simulink model "tqdtqr_rebuild_V3"  (R2021b)
settings: Solver=VariableStepAuto  StartTime=0.0  StopTime=10.0  RelTol=1e-3
undefined symbols (not defined in the file): ATQD_AfterTqMinGain_X_Deg, ATQD_APSCreepBaseTqD_X_kph, ATQD_APSCreepBaseTqD_Y_Deg, ATQD_APSCreepBaseTqR_X_kph, ATQD_APSCreepBaseTqR_Y_Deg, ATQD_APSCreepIterm_X_kph, ATQD_APSCreepIterm_Y_kph, ATQD_APSCreepPterm_X_kph, ATQD_APSCreepPterm_Y_kph, ATQD_APSDecReq_X_kph, ATQD_APSDecReq_Y_mps2, ATQD_APSDecReqCMD_X_kph, ATQD_APSDecReqTs_X_pct, ATQD_APSDecTimeGain_X_Deg, ATQD_APSDecTimeGain_Y_s, ATQD_APSReqLowSpd_X_Deg, ATQD_AutoHoldReleaseBPS_X_Deg, ATQD_AWDLoadTrqnsGain_X_kg, ATQD_AWDLoadTrqnsGain_Y_pct, ATQD_BOSEnBPSPosn_X_kph, ATQD_BOSMap_X_rpm, ATQD_BOSMap_Y_pct, ATQD_CreepBaseTqD_X_kph, ATQD_CreepBaseTqD_Y_Deg, ATQD_CreepBaseTqR_X_kph, ATQD_CreepBaseTqR_Y_Deg, ATQD_CreepBPSDisPosn_X_Deg, ATQD_CreepBPSDisPosnR_X_Deg, ATQD_CreepBPSEnPosn_X_Deg, ATQD_CreepBPSEnPosnR_X_Deg, ATQD_CreepDeltaTq_X_kph, ATQD_CreepIterm_X_kph, ATQD_CreepIterm_Y_kph, ATQD_CreepItermMaxLimit_X_pct, ATQD_CreepPreloadTime_X_kph, ATQD_CreepPreloadTq_X_kph, ATQD_CreepPreloadTq_Y_s, ATQD_CreepProtTq_X_Deg, ATQD_CreepPterm_X_kph, ATQD_CreepPterm_Y_kph, ATQD_CreepRrTqSpRat_X_rpm, ATQD_CreepRrTqSpRat_Y_Nm, ATQD_CreepTargetSpdD_X_pct, ATQD_CreepTargetSpdR_X_pct, ATQD_CreepUpLimitTq_X_rpm, ATQD_DecIneOPDHoldEnDelay_X_Deg, ATQD_DecIneOPDHoldEnDelay_Y_bar, ATQD_ECOTqMapD_X_rpm, ATQD_ECOTqMapD_Y_pct, ATQD_EMTqMapD_X_rpm, ATQD_EMTqMapD_Y_pct, ATQD_EOPDTqMapDCon_X_rpm, ATQD_EOPDTqMapDCon_Y_Deg, ATQD_EstInitVehWeight_X_c, ATQD_FAfterTqCMDGain_X_rpm, ATQD_FAfterTqCMDGain_Y_pct, ATQD_ForceLowSpd_X_Deg, ATQD_ForcePLimitSpd_X_Deg, ATQD_FrLossMAPLowV_X_rpm, ATQD_FrLossMAPLowV_Y_Nm ... (+949)
libraries: simulink x235, hcu_lib x208, tqr x63, tqd x6
(part 11 of 37)

== system tqdtqr_rebuild_V3/Input_Convert/Main function/Front//Rear zero point transfer ==
  note: Determine increase/decrease value
  note: Detemine rear zero transform
  note: Rear zero up/low boundary
  note: Detemine front zero transform
  note: Front zero up/low boundary
  BSCPIn_outputs : Inport
  BSignalConvert_outputs : Inport  Port=2
  BMain_outputs : Inport  Port=3
  VTQD_CreepPrLoadEnable_flg : Inport  Port=4
  VTQD_PreLoadPreEn_flg : Inport  Port=5
  AND : Logic  Inputs=4  AllPortsSameDT=off  OutDataTypeStr=boolean
  AND1 : Logic  Inputs=4  AllPortsSameDT=off  OutDataTypeStr=boolean
  Bus Selector : BusSelector  OutputSignals=VVMC_ADASActive_flg,VVMC_ACCPedalOvrd_flg,VVMC_EstSlope_Deg,VINP_VehSpeed_kph
  Bus Selector1 : BusSelector  OutputSignals=VTQR_EVDriveMode_enum,VTQD_TqTargetShaftSpd_rpm,VTQR_LaunchEn_flg,VTQD_RegenMode_enum
  Bus Selector2 : BusSelector  OutputSignals=VTQD_AfterAvailableTqDemFr_Nm,VTQD_AfterAvailableTqDemRr_Nm,VTQR_FEDUWhlTqReqSmoothDelay_Nm,VTQR_REDUWhlTqReqSmoothDelay_Nm
  Constant : Constant  Value=ZERO_FLOAT
  Constant{1,11,13..14} (4 alike) : Constant  Value=ENUM_DRIVEMODE_ECO
  Constant10 : Constant  Value=KTQR_OPDNoZeroTransSpd_kph
  Constant{2,12,15,18} (4 alike) : Constant  Value=ENUM_DRIVEMODE_NRM
  Constant{3,16..17,19} (4 alike) : Constant  Value=ENUM_DRIVEMODE_SPORT
  Constant20 : Constant  Value=ZERO_FLOAT
  Constant{4,21,28..29} (4 alike) : Constant  Value=ENUM_TQZEROTRANS_POSITIVE
  Constant22 : Constant  Value=ENUM_TQZEROTRANS_NEGATIVE
  Constant23 : Constant  Value=ENUM_TQZEROTRANS_NOZEROTRANS
  Constant24 : Constant  Value=KTQR_CreepZeroTransSW_flg
  Constant25 : Constant  Value=ENUM_REGENLEVEL_OPD
  Constant26 : Constant  Value=KTQR_OPDNoZeroTransTq_Nm
  Constant27 : Constant  Value=KTQR_OPDNoZeroTransSpd_kph
  Constant5 : Constant  Value=ENUM_TQZEROTRANS_NEGATIVE
  Constant6 : Constant  Value=ENUM_TQZEROTRANS_NOZEROTRANS
  Constant7 : Constant  Value=KTQR_CreepZeroTransSW_flg
  Constant8 : Constant  Value=ENUM_REGENLEVEL_OPD
  Constant9 : Constant  Value=KTQR_OPDNoZeroTransTq_Nm
  EcoLow : tqr/TQR/Determine Torque Request/TorqueArbitrament/TorqueSmooth/Front Torque zero point transfer boundary map/EcoLow  SystemSampleTime=-1  VariantActivationTime=update diagram  Latency=0  AutoFrameSizeCalculation=off
  EcoLow1 : tqr/TQR/Determine Torque Request/TorqueArbitrament/TorqueSmooth/Rear Torque zero point transfer boundary map/EcoLow  SystemSampleTime=-1  VariantActivationTime=update diagram  Latency=0  AutoFrameSizeCalculation=off
  EcoUP : tqr/TQR/Determine Torque Request/TorqueArbitrament/TorqueSmooth/Front Torque zero point transfer boundary map/EcoUP  SystemSampleTime=-1  VariantActivationTime=update diagram  Latency=0  AutoFrameSizeCalculation=off
  EcoUP1 : tqr/TQR/Determine Torque Request/TorqueArbitrament/TorqueSmooth/Rear Torque zero point transfer boundary map/EcoUP  SystemSampleTime=-1  VariantActivationTime=update diagram  Latency=0  AutoFrameSizeCalculation=off
  Equal{,1..13} (14 alike) : RelationalOperator  Operator===  OutDataTypeStr=boolean  RndMeth=Simplest
  If{1..4} (4 alike) : If  NumInputs=3  IfExpression=u1~= 0  ElseIfExpressions=u2 ~= 0, u3 ~=0  ShowElse=off
  Logical Operator : Logic  Inputs=7  AllPortsSameDT=off  OutDataTypeStr=boolean
  Logical Operator{1..4,6..9} (8 alike) : Logic  Operator=NOT  AllPortsSameDT=off  OutDataTypeStr=boolean
  Logical Operator5 : Logic  Inputs=7  AllPortsSameDT=off  OutDataTypeStr=boolean
  Merge{,1..3} (4 alike) : Merge  Inputs=3
  NOT{,1..3} (4 alike) : Logic  Operator=NOT  AllPortsSameDT=off  OutDataTypeStr=boolean
  Negative Rate limit Determination : Subsystem  TreatAsAtomicUnit=on
  Negative Rate limit Determination1 : Subsystem  AncestorBlock=tqr/TQR/Determine Torque Request/TorqueArbitrament/TorqueSmooth/Rear wheel rate limit determination/Negative Rate limit Determination  TreatAsAtomicUnit=on
  NormalLow : tqr/TQR/Determine Torque Request/TorqueArbitrament/TorqueSmooth/Front Torque zero point transfer boundary map/NormalLow  SystemSampleTime=-1  VariantActivationTime=update diagram  Latency=0  AutoFrameSizeCalculation=off
  NormalLow1 : tqr/TQR/Determine Torque Request/TorqueArbitrament/TorqueSmooth/Rear Torque zero point transfer boundary map/NormalLow  SystemSampleTime=-1  VariantActivationTime=update diagram  Latency=0  AutoFrameSizeCalculation=off
  NormalUP : tqr/TQR/Determine Torque Request/TorqueArbitrament/TorqueSmooth/Front Torque zero point transfer boundary map/NormalUP  SystemSampleTime=-1  VariantActivationTime=update diagram  Latency=0  AutoFrameSizeCalculation=off
  NormalUP1 : tqr/TQR/Determine Torque Request/TorqueArbitrament/TorqueSmooth/Rear Torque zero point transfer boundary map/NormalUP  SystemSampleTime=-1  VariantActivationTime=update diagram  Latency=0  AutoFrameSizeCalculation=off
  OR{,1..3} (4 alike) : Logic  Operator=OR  AllPortsSameDT=off  OutDataTypeStr=boolean
  Positive Rate limit Determination : Subsystem  TreatAsAtomicUnit=on
  Positive Rate limit Determination1 : Subsystem  TreatAsAtomicUnit=on
  Relational Operator : RelationalOperator  Operator=<  OutDataTypeStr=boolean  RndMeth=Simplest
  Relational Operator1 : RelationalOperator  Operator=>  OutDataTypeStr=boolean  RndMeth=Simplest
  Relational Operator10 : RelationalOperator  Operator===  OutDataTypeStr=boolean  RndMeth=Simplest
  Relational Operator11 : RelationalOperator  Operator===  OutDataTypeStr=boolean  RndMeth=Simplest
  Relational Operator2 : RelationalOperator  OutDataTypeStr=boolean  RndMeth=Simplest
  Relational Operator{3..4,8..9} (4 alike) : RelationalOperator  Operator=<=  OutDataTypeStr=boolean  RndMeth=Simplest
  Relational Operator5 : RelationalOperator  Operator=<  OutDataTypeStr=boolean  RndMeth=Simplest
  Relational Operator6 : RelationalOperator  Operator=>  OutDataTypeStr=boolean  RndMeth=Simplest
  Relational Operator7 : RelationalOperator  OutDataTypeStr=boolean  RndMeth=Simplest
  Relay1 : Relay  OnSwitchValue=KTQD_OPDHoldGradeUp_Deg  OffSwitchValue=KTQD_OPDHoldGradeDown_Deg  OutDataTypeStr=boolean
      settings: AttributesFormatString=|
      | On : %<OnSwitchValue>
      | Off : %<OffSwitchValue>
  Relay2 : Relay  OnSwitchValue=KTQD_OPDHoldGradeUp_Deg  OffSwitchValue=KTQD_OPDHoldGradeDown_Deg  OutDataTypeStr=boolean
      settings: AttributesFormatString=|
      | Off: %<OffOutputValue>
      | On: %<OnSwitchValue>
  SportLow : tqr/TQR/Determine Torque Request/TorqueArbitrament/TorqueSmooth/Front Torque zero point transfer boundary map/SportLow  SystemSampleTime=-1  VariantActivationTime=update diagram  Latency=0  AutoFrameSizeCalculation=off
  SportLow1 : tqr/TQR/Determine Torque Request/TorqueArbitrament/TorqueSmooth/Rear Torque zero point transfer boundary map/SportLow  SystemSampleTime=-1  VariantActivationTime=update diagram  Latency=0  AutoFrameSizeCalculation=off
  SportUP : tqr/TQR/Determine Torque Request/TorqueArbitrament/TorqueSmooth/Front Torque zero point transfer boundary map/SportUP  SystemSampleTime=-1  VariantActivationTime=update diagram  Latency=0  AutoFrameSizeCalculation=off
  SportUP1 : tqr/TQR/Determine Torque Request/TorqueArbitrament/TorqueSmooth/Rear Torque zero point transfer boundary map/SportUP  SystemSampleTime=-1  VariantActivationTime=update diagram  Latency=0  AutoFrameSizeCalculation=off
  Switch{,1..3} (4 alike) : Switch  Criteria=u2 ~= 0
      settings: AttributesFormatString=%<Criteria>
  Switch4 : Switch  Criteria=u2 ~= 0  Threshold=0.5
      settings: AttributesFormatString=%<Criteria>
  Switch5 : Switch  Criteria=u2 ~= 0  Threshold=0.5
      settings: AttributesFormatString=%<Criteria>
  VTQR_FrTqZeroTransUpBound_Nm : Outport
  VTQR_FrTqZeroTransLowBound_Nm : Outport  Port=2
  VTQR_FrTqZeroTrans_enum : Outport  Port=3
  VTQR_RrTqZeroTransUpBound_Nm : Outport  Port=4
  VTQR_RrTqZeroTransLowBound_Nm : Outport  Port=5
  VTQR_RrTqZeroTrans_enum : Outport  Port=6
  VTQD_FrZeroPointIncDec_Nm : Outport  Port=7
  VTQD_RrZeroPointIncDec_Nm : Outport  Port=8
  wires:
  If2/2 -> EcoLow/Action
  NormalLow/1 -> Merge1/1
  Constant12/1 -> Equal11/2
  If2/3 -> SportLow/Action
  Constant2/1 -> Equal4/2
  Equal5/1 -> If2/3
  [VTQR_EVDriveMode_enum] -> Equal5/1
  If2/1 -> NormalLow/Action
  If1/3 -> SportUP/Action
  Merge/1 -> [VTQR_FrTqZeroTransUpBound_Nm]  "VTQR_FrTqZeroTransUpBound_Nm"
  Constant11/1 -> Equal1/2
  Merge1/1 -> [VTQR_FrTqZeroTransLowBound_Nm]  "VTQR_FrTqZeroTransLowBound_Nm"
  Equal1/1 -> If1/2
  [VTQD_TqTargetShaftSpd_rpm] -> SportLow/1
  If1/2 -> EcoUP/Action
  [VTQR_EVDriveMode_enum] -> Equal4/1
  Constant1/1 -> Equal3/2
  [VTQR_EVDriveMode_enum] -> Equal3/1
  SportLow/1 -> Merge1/3
  Constant16/1 -> Equal2/2
  [VTQR_EVDriveMode_enum] -> Equal1/1
  Equal4/1 -> If2/1
  [VTQD_TqTargetShaftSpd_rpm] -> EcoLow/1
  [VTQD_TqTargetShaftSpd_rpm] -> NormalLow/1
  Equal2/1 -> If1/3
  NormalUP/1 -> Merge/1
  [VTQD_TqTargetShaftSpd_rpm] -> SportUP/1
  [VTQR_EVDriveMode_enum] -> Equal11/1
  EcoLow/1 -> Merge1/2
  SportUP/1 -> Merge/3
  Equal3/1 -> If2/2
  If1/1 -> NormalUP/Action
  [VTQD_TqTargetShaftSpd_rpm] -> NormalUP/1
  Equal11/1 -> If1/1
  [VTQD_TqTargetShaftSpd_rpm] -> EcoUP/1
  Constant3/1 -> Equal5/2
  [VTQR_EVDriveMode_enum] -> Equal2/1
  EcoUP/1 -> Merge/2
  Constant5/1 -> Switch1/3
  [VTQR_FEDUWhlTqReqSmoothDelay_Nm] -> Relational Operator/1
  [VTQR_LaunchEn_flg] -> Logical Operator4/1
  Relational Operator2/1 -> Switch1/2
  Logical Operator/1 -> Switch/2
  Logical Operator3/1 -> Logical Operator/5
  Relational Operator1/1 -> Logical Operator/2
  [VVMC_ACCPedalOvrd_flg] -> OR/2
  Logical Operator2/1 -> OR/1
  [VTQR_FrTqZeroTransLowBound_Nm] -> Relational Operator1/2
  [VINP_VehSpeed_kph] -> Relational Operator4/1
  [VVMC_ADASActive_flg] -> Logical Operator2/1
  Switch1/1 -> Switch/1
  Relational Operator/1 -> Logical Operator/1
  [VVMC_EstSlope_Deg] -> Relay1/1
  Relational Operator4/1 -> AND/4
  [VTQD_RegenMode_enum] -> Equal/1
  Equal/1 -> AND/2
  OR1/1 -> Logical Operator/3
  [VTQR_FEDUWhlTqReqSmoothDelay_Nm] -> Relational Operator2/1
  [VTQD_AfterAvailableTqDemFr_Nm] -> Relational Operator3/1
  Relay1/1 -> NOT3/1
  Switch/1 -> [VTQR_FrTqZeroTrans_enum]  "VTQR_FrTqZeroTrans_enum"
  AND/1 -> NOT/1
  [VTQR_FEDUWhlTqReqSmoothDelay_Nm] -> Relational Operator1/1
  OR/1 -> Logical Operator/4
  [VTQR_FrTqZeroTransUpBound_Nm] -> Relational Operator/2
  Relational Operator3/1 -> AND/3
  NOT/1 -> Logical Operator/7
  Constant6/1 -> Switch/3
  Constant4/1 -> Switch1/1
  [VTQD_PreLoadPreEn_flg] -> Logical Operator3/1
  Constant9/1 -> Relational Operator3/2
  Logical Operator4/1 -> Logical Operator/6
  [VTQD_CreepPrLoadEnable_flg] -> Logical Operator1/1
  Constant10/1 -> Relational Operator4/2
  NOT3/1 -> AND/1
  Constant/1 -> Relational Operator2/2
  Logical Operator1/1 -> OR1/1
  Constant7/1 -> OR1/2
  Constant8/1 -> Equal/2
  BSCPIn_outputs/1 -> Bus Selector/1
  BSignalConvert_outputs/1 -> Bus Selector1/1
  BMain_outputs/1 -> Bus Selector2/1
  Bus Selector1/1 -> [VTQR_EVDriveMode_enum]  "<VTQR_EVDriveMode_enum>"
  Bus Selector1/2 -> [VTQD_TqTargetShaftSpd_rpm]  "<VTQD_TqTargetShaftSpd_rpm>"
  VTQD_CreepPrLoadEnable_flg/1 -> [VTQD_CreepPrLoadEnable_flg]
  Bus Selector/1 -> [VVMC_ADASActive_flg]  "<VVMC_ADASActive_flg>"
  Bus Selector/2 -> [VVMC_ACCPedalOvrd_flg]  "<VVMC_ACCPedalOvrd_flg>"
  VTQD_PreLoadPreEn_flg/1 -> [VTQD_PreLoadPreEn_flg]
  Bus Selector1/3 -> [VTQR_LaunchEn_flg]  "<VTQR_LaunchEn_flg>"
  Bus Selector/3 -> [VVMC_EstSlope_Deg]  "<VVMC_EstSlope_Deg>"
  Bus Selector1/4 -> [VTQD_RegenMode_enum]  "<VTQD_RegenMode_enum>"
  Bus Selector2/1 -> [VTQD_AfterAvailableTqDemFr_Nm]  "<VTQD_AfterAvailableTqDemFr_Nm>"
  Bus Selector/4 -> [VINP_VehSpeed_kph]  "<VINP_VehSpeed_kph>"
  [VTQR_FrTqZeroTransUpBound_Nm] -> VTQR_FrTqZeroTransUpBound_Nm/1
  [VTQR_FrTqZeroTransLowBound_Nm] -> VTQR_FrTqZeroTransLowBound_Nm/1
  [VTQR_FrTqZeroTrans_enum] -> VTQR_FrTqZeroTrans_enum/1
  SportUP1/1 -> Merge2/3
  EcoLow1/1 -> Merge3/2
  [VTQR_EVDriveMode_enum] -> Equal12/1
  Constant18/1 -> Equal10/2
  NormalLow1/1 -> Merge3/1
  [VTQR_EVDriveMode_enum] -> Equal10/1
  Equal10/1 -> If4/1
  Merge3/1 -> [VTQR_RrTqZeroTransLowBound_Nm]  "VTQR_RrTqZeroTransLowBound_Nm"
  [VTQR_EVDriveMode_enum] -> Equal6/1
  [VTQR_EVDriveMode_enum] -> Equal9/1
  SportLow1/1 -> Merge3/3
  Constant17/1 -> Equal8/2
  Equal7/1 -> If3/1
  [VTQD_TqTargetShaftSpd_rpm] -> NormalLow1/1
  Equal8/1 -> If3/3
  [VTQR_EVDriveMode_enum] -> Equal8/1
  Constant19/1 -> Equal12/2
  Constant14/1 -> Equal6/2
  Constant15/1 -> Equal7/2
  Constant13/1 -> Equal9/2
  Merge2/1 -> [VTQR_RrTqZeroTransUpBound_Nm]  "VTQR_RrTqZeroTransUpBound_Nm"
  If4/3 -> SportLow1/Action
  If4/2 -> EcoLow1/Action
  [VTQR_EVDriveMode_enum] -> Equal7/1
  If4/1 -> NormalLow1/Action
  [VTQD_TqTargetShaftSpd_rpm] -> EcoLow1/1
  Equal12/1 -> If4/3
  Equal6/1 -> If3/2
  If3/2 -> EcoUP1/Action
  [VTQD_TqTargetShaftSpd_rpm] -> SportUP1/1
  EcoUP1/1 -> Merge2/2
  NormalUP1/1 -> Merge2/1
  If3/3 -> SportUP1/Action
  [VTQD_TqTargetShaftSpd_rpm] -> SportLow1/1
  Equal9/1 -> If4/2
  If3/1 -> NormalUP1/Action
  [VTQD_TqTargetShaftSpd_rpm] -> EcoUP1/1
  [VTQD_TqTargetShaftSpd_rpm] -> NormalUP1/1
  [VTQR_REDUWhlTqReqSmoothDelay_Nm] -> Relational Operator7/1
  Constant20/1 -> Relational Operator7/2
  Constant26/1 -> Relational Operator8/2
  [VTQR_REDUWhlTqReqSmoothDelay_Nm] -> Relational Operator6/1
  Relational Operator5/1 -> Logical Operator5/1
  [VTQR_RrTqZeroTransLowBound_Nm] -> Relational Operator6/2
  Equal13/1 -> AND1/2
  [VTQR_LaunchEn_flg] -> Logical Operator9/1
  [VVMC_ADASActive_flg] -> Logical Operator7/1
  [VINP_VehSpeed_kph] -> Relational Operator9/1
  [VTQD_PreLoadPreEn_flg] -> Logical Operator8/1
  [VTQR_RrTqZeroTransUpBound_Nm] -> Relational Operator5/2
  NOT1/1 -> Logical Operator5/7
  NOT2/1 -> AND1/1
  OR2/1 -> Logical Operator5/4
  Constant27/1 -> Relational Operator9/2
  [VTQD_RegenMode_enum] -> Equal13/1
  [VVMC_EstSlope_Deg] -> Relay2/1
  Relational Operator9/1 -> AND1/4
  Constant22/1 -> Switch3/3
  Relational Operator6/1 -> Logical Operator5/2
  Logical Operator5/1 -> Switch2/2
  Constant25/1 -> Equal13/2
  Relay2/1 -> NOT2/1
  [VTQR_REDUWhlTqReqSmoothDelay_Nm] -> Relational Operator5/1
  Logical Operator6/1 -> OR3/1
  Constant21/1 -> Switch3/1
  Switch2/1 -> [VTQR_RrTqZeroTrans_enum]  "VTQR_RrTqZeroTrans_enum"
  AND1/1 -> NOT1/1
  Switch3/1 -> Switch2/1
  OR3/1 -> Logical Operator5/3
  Constant24/1 -> OR3/2
  Logical Operator7/1 -> OR2/1
  [VTQD_CreepPrLoadEnable_flg] -> Logical Operator6/1
  Relational Operator7/1 -> Switch3/2
  [VVMC_ACCPedalOvrd_flg] -> OR2/2
  Logical Operator9/1 -> Logical Operator5/6
  Constant23/1 -> Switch2/3
  Logical Operator8/1 -> Logical Operator5/5
  [VTQD_AfterAvailableTqDemRr_Nm] -> Relational Operator8/1
  Relational Operator8/1 -> AND1/3
  Bus Selector2/2 -> [VTQD_AfterAvailableTqDemRr_Nm]  "<VTQD_AfterAvailableTqDemRr_Nm>"
  [VTQR_RrTqZeroTransUpBound_Nm] -> VTQR_RrTqZeroTransUpBound_Nm/1
  [VTQR_RrTqZeroTransLowBound_Nm] -> VTQR_RrTqZeroTransLowBound_Nm/1
  [VTQR_RrTqZeroTrans_enum] -> VTQR_RrTqZeroTrans_enum/1
  Bus Selector2/3 -> [VTQR_FEDUWhlTqReqSmoothDelay_Nm]  "<VTQR_FEDUWhlTqReqSmoothDelay_Nm>"
  Bus Selector2/4 -> [VTQR_REDUWhlTqReqSmoothDelay_Nm]  "<VTQR_REDUWhlTqReqSmoothDelay_Nm>"
  [VTQR_FEDUWhlTqReqSmoothDelay_Nm] -> Negative Rate limit Determination/2(VTQR_FEDUWhlTqReqSmoothDelay_Nm)
  [VTQR_EVDriveMode_enum] -> Negative Rate limit Determination/3(VTQR_EVDriveMode_enum)
  [VTQR_EVDriveMode_enum] -> Positive Rate limit Determination/3(VTQR_EVDriveMode_enum)
  [VTQD_TqTargetShaftSpd_rpm] -> Positive Rate limit Determination/1(VTQD_TqTargetShaftSpd_rpm)
  [VTQR_FEDUWhlTqReqSmoothDelay_Nm] -> Positive Rate limit Determination/2(VTQR_FEDUWhlTqReqSmoothDelay_Nm)
  Relational Operator10/1 -> Switch4/2
  Negative Rate limit Determination/1(VTQR_NegRateLimit_mux) -> Switch4/3
  [VTQR_FrTqZeroTrans_enum] -> Relational Operator10/1
  Positive Rate limit Determination/1(VTQR_PosRateLimit_mux) -> Switch4/1
  [VTQD_TqTargetShaftSpd_rpm] -> Negative Rate limit Determination/1(VTQD_TqTargetShaftSpd_rpm)
  Constant28/1 -> Relational Operator10/2
  Switch4/1 -> [VTQD_FrZeroPointIncDec_Nm]
  [VTQR_RrTqZeroTrans_enum] -> Relational Operator11/1
  [VTQR_REDUWhlTqReqSmoothDelay_Nm] -> Positive Rate limit Determination1/2(VTQR_REDUWhlTqReqSmoothDelay_Nm)
  [VTQR_REDUWhlTqReqSmoothDelay_Nm] -> Negative Rate limit Determination1/2(VTQR_REDUWhlTqReqSmoothDelay_Nm)
  [VTQD_TqTargetShaftSpd_rpm] -> Negative Rate limit Determination1/1(VTQD_TqTargetShaftSpd_rpm)
  Relational Operator11/1 -> Switch5/2
  Constant29/1 -> Relational Operator11/2
  Positive Rate limit Determination1/1(VTQR_PosRateLimit_mux) -> Switch5/1
  [VTQR_EVDriveMode_enum] -> Negative Rate limit Determination1/3(VTQR_EVDriveMode_enum)
  [VTQD_TqTargetShaftSpd_rpm] -> Positive Rate limit Determination1/1(VTQD_TqTargetShaftSpd_rpm)
  Negative Rate limit Determination1/1(VTQR_NegRateLimit_mux) -> Switch5/3
  [VTQR_EVDriveMode_enum] -> Positive Rate limit Determination1/3(VTQR_EVDriveMode_enum)
  Switch5/1 -> [VTQD_RrZeroPointIncDec_Nm]
  [VTQD_FrZeroPointIncDec_Nm] -> VTQD_FrZeroPointIncDec_Nm/1
  [VTQD_RrZeroPointIncDec_Nm] -> VTQD_RrZeroPointIncDec_Nm/1

== system tqdtqr_rebuild_V3/Input_Convert/Main function/Gear detection to inverse motor ==
  note: Rear gear detect
  note: Front gear detect
  BFunction_outputs : Inport
  BMain_outputs : Inport  Port=2
  Abs : Abs
  Abs1 : Abs
  Bus Selector : BusSelector  OutputSignals=VTQD_GearActualPosn_enum
  Bus Selector1 : BusSelector  OutputSignals=VTQR_FrTMTqReq_Nm,VTQR_RrTMTqReq_Nm
  Constant20 : Constant  Value=KTQR_GearEnChangeTq_Nm
  Constant22 : Constant  Value=KTQR_GearEnChangeTq_Nm
  Delay4 : Delay  DelayLength=1  InitialCondition=single(0)
      settings: AttributesFormatString=%<InitialCondition>
  Delay5 : Delay  DelayLength=1  InitialCondition=single(0)
      settings: AttributesFormatString=%<InitialCondition>
  Detect Change : simulink/Logic and Bit Operations/Detect Change  vinit=0  OutDataTypeStr=boolean
  Detect Change1 : simulink/Logic and Bit Operations/Detect Change  vinit=0  OutDataTypeStr=boolean
  Relational Operator4 : RelationalOperator  Operator=<=  OutDataTypeStr=boolean  RndMeth=Simplest
  Relational Operator5 : RelationalOperator  Operator=<=  OutDataTypeStr=boolean  RndMeth=Simplest
  SR_Latch : hcu_lib/Basic_Blocks/SR_Latch
  SR_Latch1 : hcu_lib/Basic_Blocks/SR_Latch
  VTQR_FrGearChange_flg : Outport
  VTQR_RrGearChange_flg : Outport  Port=2
  wires:
  [VTQR_FrTMTqReq_Nm] -> Delay4/1
  Abs/1 -> Relational Operator4/1
  [VTQD_GearActualPosn_enum] -> Detect Change/1
  Delay4/1 -> Abs/1
  Relational Operator4/1 -> SR_Latch/2
  Constant20/1 -> Relational Operator4/2
  Detect Change/1 -> SR_Latch/1
  SR_Latch/1 -> [VTQR_FrGearChange_flg]  "VTQR_FrGearChange_flg"
  Abs1/1 -> Relational Operator5/1
  [VTQR_RrTMTqReq_Nm] -> Delay5/1
  Detect Change1/1 -> SR_Latch1/1
  Relational Operator5/1 -> SR_Latch1/2
  Constant22/1 -> Relational Operator5/2
  Delay5/1 -> Abs1/1
  SR_Latch1/1 -> [VTQR_RrGearChange_flg]  "VTQR_RrGearChange_flg"
  [VTQD_GearActualPosn_enum] -> Detect Change1/1
  BFunction_outputs/1 -> Bus Selector/1
  Bus Selector/1 -> [VTQD_GearActualPosn_enum]  "<VTQD_GearActualPosn_enum>"
  [VTQR_FrGearChange_flg] -> VTQR_FrGearChange_flg/1
  [VTQR_RrGearChange_flg] -> VTQR_RrGearChange_flg/1
  BMain_outputs/1 -> Bus Selector1/1
  Bus Selector1/1 -> [VTQR_FrTMTqReq_Nm]  "<VTQR_FrTMTqReq_Nm>"
  Bus Selector1/2 -> [VTQR_RrTMTqReq_Nm]  "<VTQR_RrTMTqReq_Nm>"

== system tqdtqr_rebuild_V3/Input_Convert/Main function/Tq coordination function ==
  note: Determine Tq source
  note: Total Comman Capacity Torque
  note: HV Available Output Torque Power
  note: Determine Fr/Rr torque source
  BSCPIn_outputs : Inport
  BSignalConvert_outputs : Inport  Port=2
  BMain_outputs : Inport  Port=3
  VTQD_RollRegenEnable_flg : Inport  Port=4
  VTQD_MotorLossTotal_kw : Inport  Port=5
  AND2 : Logic  Inputs=5  AllPortsSameDT=off  OutDataTypeStr=boolean
  AND3 : Logic  Operator=OR  AllPortsSameDT=off  OutDataTypeStr=boolean
  AND4 : Logic  Inputs=5  AllPortsSameDT=off  OutDataTypeStr=boolean
  AND5 : Logic  Operator=OR  AllPortsSameDT=off  OutDataTypeStr=boolean
  Abs{,1..6} (7 alike) : Abs
  Add : Sum
  Bus Selector : BusSelector  OutputSignals=VINP_HVBPwrAvailDchrg_kW,VINP_HVBPwrAvailChrg_kW,VVMC_ADASForceIdle_flg,VVMC_ADASActive_flg,VVMC_CruzActive_flg,VVMC_MSAActive_flg,VVMC_APSActive_flg,VINP_FrRBCActive_flg,VINP_RrRBCActive_flg,VINP_VehSpeed_kph
  Bus Selector1 : BusSelector  OutputSignals=VTQD_FrShaftSpd_rpm,VTQD_RrShaftSpd_rpm,VTQD_NoSuitbleGear_flg
  Bus Selector2 : BusSelector  OutputSignals=VTQD_DriverWhlTqDem_Nm,VTQD_CoordTqDem_Nm
  Constant : Constant  Value=KTQD_DCDCCalPwrAvailRsv_kW
  Constant1 : Constant  Value=KTQD_THCMCalPwrAvailRsv_kW
  Constant10 : Constant  Value=ENUM_TQSOURCE_ADAS
  Constant11 : Constant  Value=ENUM_TQSOURCE_CC
  Constant12 : Constant  Value=ENUM_TQSOURCE_MSA
  Constant13 : Constant  Value=ENUM_TQSOURCE_APS
  Constant14 : Constant  Value=ENUM_TQSOURCE_INTERNAL
  Constant15 : Constant  Value=ENUM_TQSOURCE_INVALID  VectorParams1D=off  SampleTime=-1
  Constant16 : Constant  Value=ZERO_FLOAT  VectorParams1D=off  SampleTime=-1
  Constant17 : Constant  Value=ENUM_TQSOURCE_ABS  VectorParams1D=off  SampleTime=-1
  Constant18 : Constant  Value=ENUM_TQSOURCE_INVALID  VectorParams1D=off  SampleTime=-1
  Constant19 : Constant  Value=ZERO_FLOAT  VectorParams1D=off  SampleTime=-1
  Constant2 : Constant  Value=KTQD_TMPwrAvailDchrg_kW_ovrdflg
  Constant20 : Constant  Value=ENUM_TQSOURCE_ABS  VectorParams1D=off  SampleTime=-1
  Constant21 : Constant  Value=ENUM_TQSOURCE_ROLLABS  VectorParams1D=off  SampleTime=-1
  Constant22 : Constant  Value=ENUM_TQSOURCE_ADAS  VectorParams1D=off  SampleTime=-1
  Constant23 : Constant  Value=ENUM_TQSOURCE_ADAS  VectorParams1D=off  SampleTime=-1
  Constant24 : Constant  Value=ENUM_TQSOURCE_CC  SampleTime=-1
  Constant25 : Constant  Value=ENUM_TQSOURCE_MSA  SampleTime=-1
  Constant26 : Constant  Value=ENUM_TQSOURCE_CC  SampleTime=-1
  Constant27 : Constant  Value=ENUM_TQSOURCE_MSA  SampleTime=-1
  Constant28 : Constant  Value=ENUM_TQSOURCE_ROLLABS  VectorParams1D=off  SampleTime=-1
  Constant29 : Constant  Value=KTQD_AEBEmergBrkSpd_kph
  Constant3 : Constant  Value=ZERO_FLOAT
  Constant30 : Constant  Value=ZERO_FLOAT
  Constant4 : Constant  Value=KTQD_BatapCont_factor
  Constant5 : Constant  Value=ONE_FLOAT
  Constant6 : Constant  Value=KTQD_BatapCont_factor
  Constant7 : Constant  Value=ONE_FLOAT
  Constant8 : Constant  Value=ENUM_TQSOURCE_INVALID
  Constant9 : Constant  Value=ENUM_TQSOURCE_ADASFORCEIDLE
  Data Type Conversion2 : DataTypeConversion  OutDataTypeStr=uint8
  Delay : Delay  DelayLength=1  InitialCondition=single(0)
      settings: AttributesFormatString=%<InitialCondition>
  Delay1 : Delay  DelayLength=1  InitialCondition=single(0)
      settings: AttributesFormatString=%<InitialCondition>
  Delay2 : Delay  DelayLength=1  InitialCondition=single(0)
      settings: AttributesFormatString=%<InitialCondition>
  Equal{,6,8..13} (8 alike) : RelationalOperator  Operator=~=  OutDataTypeStr=boolean  RndMeth=Simplest
  Equal5 : RelationalOperator  Operator=<  OutDataTypeStr=boolean  RndMeth=Simplest
  Equal7 : RelationalOperator  Operator=<  OutDataTypeStr=boolean  RndMeth=Simplest
  Fcn : Fcn  Expr=u[1]/u[2]/pi*u[3]
  Fcn1 : Fcn  Expr=u[1]/u[2]/pi*u[3]
  Gain4 : Gain  Gain=MINUSONE_FLOAT
  Max : MinMax  Function=max  Inputs=2
  Max1 : MinMax  Function=max  Inputs=3
  Max2 : MinMax  Function=max  Inputs=3
  Mux : Mux  Inputs=3
  Mux1 : Mux  Inputs=3
  Relational Operator : RelationalOperator  Operator=<  OutDataTypeStr=boolean  RndMeth=Simplest
  Saturation : Saturate  UpperLimit=ZERO_FLOAT  LowerLimit=KTQD_ForceIdleRgnLim_Nm
      settings: AttributesFormatString=|
      | Up:%<UpperLimit>
      | Low:%<LowerLimit>
  Saturation1 : Saturate  UpperLimit=ZERO_FLOAT  LowerLimit=KTQD_TotalLowTheldTrq_Nm
      settings: AttributesFormatString=|
      | Upper Limit :%<UpperLimit>
      | Lower Limit :%<LowerLimit>
  Saturation2 : Saturate  UpperLimit=KTQD_TotalUpTheldTrq_Nm  LowerLimit=ZERO_FLOAT
      settings: AttributesFormatString=|
      | Upper Limit :%<UpperLimit>
      | Lower Limit :%<LowerLimit>
  Subtract : Sum  Inputs=+--
  Switch{,1..7,9,11..12} (11 alike) : Switch  Criteria=u2 ~= 0
      settings: AttributesFormatString=%<Criteria>
  Switch10 : Switch  Criteria=u2 > Threshold
  Switch8 : Switch  Criteria=u2 > Threshold
  VTQD_TqSourceFr_enum : Outport
  VTQD_TqSourceRr_enum : Outport  Port=2
  VTQD_TotalWhlTqCapMot_Nm : Outport  Port=3
  VTQD_TotalWhlTqCapGen_Nm : Outport  Port=4
  VTQD_ForceIdleTqReq_Nm : Outport  Port=5
  wires:
  Constant1/1 -> Add/2
  Subtract/1 -> Max/1
  Max/1 -> Switch/1
  Constant/1 -> Add/1
  Saturation2/1 -> [VTQD_TotalWhlTqCapMot_Nm]  "VTQD_TotalWhlTqCapMot_Nm"
  [VINP_HVBPwrAvailDchrg_kW] -> Abs/1
  [VTQD_FrShaftSpd_rpm] -> Abs2/1
  Constant3/1 -> Max/2
  Abs6/1 -> Mux1/1
  Abs2/1 -> Max1/1
  Fcn1/1 -> Gain4/1
  Abs5/1 -> Max2/2
  Mux1/1 -> Fcn1/1
  Abs3/1 -> Max1/2
  [VTQD_RrShaftSpd_rpm] -> Abs5/1
  Constant7/1 -> Max2/3
  Mux/1 -> Fcn/1
  Abs4/1 -> Max2/1
  Switch/1 -> [VTQD_TotalAvailDchrg_kW]  "VTQD_TotalAvailDchrg_kW"
  Fcn/1 -> Saturation2/1
  Constant6/1 -> Mux1/3
  Max2/1 -> Mux1/2
  [VINP_HVBPwrAvailDchrg_kW] -> Abs1/1
  [VTQD_FrShaftSpd_rpm] -> Abs4/1
  [VTQD_TotalAvailDchrg_kW] -> Mux/1
  [VINP_HVBPwrAvailChrg_kW] -> Abs6/1
  [VTQD_RrShaftSpd_rpm] -> Abs3/1
  Constant2/1 -> Switch/2
  Add/1 -> Subtract/2
  Abs1/1 -> Switch/3
  Delay/1 -> Subtract/3
  Constant5/1 -> Max1/3
  Max1/1 -> Mux/2
  [VTQD_MotorLossTotal_kw] -> Delay/1
  Abs/1 -> Subtract/1
  Gain4/1 -> Saturation1/1
  Constant4/1 -> Mux/3
  Saturation1/1 -> [VTQD_TotalWhlTqCapGen_Nm]  "VTQD_TotalWhlTqCapGen_Nm"
  BSCPIn_outputs/1 -> Bus Selector/1
  BSignalConvert_outputs/1 -> Bus Selector1/1
  Bus Selector/1 -> [VINP_HVBPwrAvailDchrg_kW]  "<VINP_HVBPwrAvailDchrg_kW>"
  Bus Selector/2 -> [VINP_HVBPwrAvailChrg_kW]  "<VINP_HVBPwrAvailChrg_kW>"
  Bus Selector1/1 -> [VTQD_FrShaftSpd_rpm]  "<VTQD_FrShaftSpd_rpm>"
  Bus Selector1/2 -> [VTQD_RrShaftSpd_rpm]  "<VTQD_RrShaftSpd_rpm>"
  [VTQD_TotalWhlTqCapMot_Nm] -> VTQD_TotalWhlTqCapMot_Nm/1
  [VTQD_TotalWhlTqCapGen_Nm] -> VTQD_TotalWhlTqCapGen_Nm/1
  Bus Selector1/3 -> [VTQD_NoSuitbleGear_flg]  "<VTQD_NoSuitbleGear_flg>"
  Bus Selector/3 -> [VINP_ADASForceIdle_flg]  "<VVMC_ADASForceIdle_flg>"
  Bus Selector/4 -> [VVMC_ADASActive_flg]  "<VVMC_ADASActive_flg>"
  Bus Selector/5 -> [VVMC_CruzActive_flg]  "<VVMC_CruzActive_flg>"
  Bus Selector/6 -> [VVMC_MSAActive_flg]  "<VVMC_MSAActive_flg>"
  Bus Selector/7 -> [VVMC_APSActive_flg]  "<VVMC_APSActive_flg>"
  [VTQD_NoSuitbleGear_flg] -> Switch1/2
  Constant8/1 -> Switch1/1
  [VINP_ADASForceIdle_flg] -> Switch2/2
  Switch2/1 -> Switch1/3
  Constant9/1 -> Switch2/1
  Switch3/1 -> Switch2/3
  [VVMC_ADASActive_flg] -> Switch3/2
  Constant10/1 -> Switch3/1
  Switch4/1 -> Switch3/3
  [VVMC_CruzActive_flg] -> Switch4/2
  Constant11/1 -> Switch4/1
  Switch5/1 -> Switch4/3
  [VVMC_MSAActive_flg] -> Switch5/2
  Constant12/1 -> Switch5/1
  Switch6/1 -> Switch5/3
  [VVMC_APSActive_flg] -> Switch6/2
  Constant13/1 -> Switch6/1
  Constant14/1 -> Switch6/3
  Switch1/1 -> Data Type Conversion2/1
  Data Type Conversion2/1 -> [VTQD_TqSource_enum]  "VTQD_TqSource_enum"
  Switch10/1 -> Switch9/1
  Equal9/1 -> AND2/1
  Switch7/1 -> [VTQD_TqSourceFr_enum]  "VTQD_TqSourceFr_enum"
  Switch9/1 -> [VTQD_TqSourceRr_enum]  "VTQD_TqSourceRr_enum"
  [VTQD_TqSource_enum] -> Equal9/1
  [VTQD_DriverWhlTqDem_Nm] -> Equal7/1
  [VINP_FrRBCActive_flg] -> AND2/3
  Equal10/1 -> AND4/2
  Equal5/1 -> AND3/1
  [VTQD_DriverWhlTqDem_Nm] -> Equal5/1
  [VTQD_TqSource_enum] -> Equal12/1
  Constant18/1 -> Equal6/2
  Equal/1 -> AND2/4
  [VTQD_TqSource_enum] -> Equal11/1
  Constant17/1 -> Switch8/3
  Switch8/1 -> Switch7/1
  Constant28/1 -> Switch8/1
  Constant16/1 -> Equal5/2
  Constant26/1 -> Equal12/2
  Constant19/1 -> Equal7/2
  Constant23/1 -> Equal9/2
  [VTQD_TqSource_enum] -> Equal10/1
  Equal12/1 -> AND2/2
  Constant15/1 -> Equal/2
  AND2/1 -> Switch7/2
  Equal13/1 -> AND2/5
  Constant22/1 -> Equal8/2
  Equal11/1 -> AND4/3
  [VTQD_TqSource_enum] -> Equal6/1
  [VTQD_TqSource_enum] -> Equal13/1
  Constant25/1 -> Equal11/2
  Equal6/1 -> AND4/5
  AND4/1 -> Switch9/2
  [VTQD_RollRegenEnable_flg] -> AND3/2
  Equal8/1 -> AND4/1
  Constant27/1 -> Equal13/2
  [VTQD_TqSource_enum] -> Switch9/3
  [VTQD_RollRegenEnable_flg] -> AND5/2
  [VTQD_TqSource_enum] -> Equal/1
  Constant24/1 -> Equal10/2
  Constant20/1 -> Switch10/3
  [VINP_RrRBCActive_flg] -> AND4/4
  [VTQD_TqSource_enum] -> Switch7/3
  [VTQD_TqSource_enum] -> Equal8/1
  AND3/1 -> Switch8/2
  AND5/1 -> Switch10/2
  Constant21/1 -> Switch10/1
  Equal7/1 -> AND5/1
  BMain_outputs/1 -> Bus Selector2/1
  Bus Selector2/1 -> [VTQD_DriverWhlTqDem_Nm]  "<VTQD_DriverWhlTqDem_Nm>"
  Bus Selector/8 -> [VINP_FrRBCActive_flg]  "<VINP_FrRBCActive_flg>"
  Bus Selector/9 -> [VINP_RrRBCActive_flg]  "<VINP_RrRBCActive_flg>"
  [VTQD_TqSourceFr_enum] -> VTQD_TqSourceFr_enum/1
  [VTQD_TqSourceRr_enum] -> VTQD_TqSourceRr_enum/1
  VTQD_RollRegenEnable_flg/1 -> [VTQD_RollRegenEnable_flg]
  VTQD_MotorLossTotal_kw/1 -> [VTQD_MotorLossTotal_kw]
  Saturation/1 -> Switch11/3
  [VINP_ADASForceIdle_flg] -> Switch11/2
  Delay1/1 -> Saturation/1
  Constant30/1 -> Switch12/1
  [VTQD_ForceIdleTqReq_Nm] -> Delay2/1
  [VINP_VehSpeed_kph] -> Relational Operator/1
  Delay2/1 -> Switch11/1
  Switch12/1 -> [VTQD_ForceIdleTqReq_Nm]  "VTQD_ForceIdleTqReq_Nm"
  Relational Operator/1 -> Switch12/2
  [VTQD_CoordTqDem_Nm] -> Delay1/1
  Constant29/1 -> Relational Operator/2
  Switch11/1 -> Switch12/3
  [VTQD_ForceIdleTqReq_Nm] -> VTQD_ForceIdleTqReq_Nm/1
  Bus Selector/10 -> [VINP_VehSpeed_kph]  "<VINP_VehSpeed_kph>"
  Bus Selector2/2 -> [VTQD_CoordTqDem_Nm]  "<VTQD_CoordTqDem_Nm>"

== system tqdtqr_rebuild_V3/Input_Convert/Main function/Tq distribution function ==
  note: New distrubution Rr/Fr torque and rate
  note: Calculate rock mode torque with Fr/Rr speed
  note: Calculate Rear ratio with Fr/Rr slide rate
  note: Fr/Rr ratio distribution
  note: AWD Rear Torque Ratio Map
  note: initia:2000kg
  note: Determine Fr/Rr rate
  BSCPIn_outputs : Inport
  BMain_outputs : Inport  Port=2
  BSignalConvert_outputs : Inport  Port=3
  BFunction_outputs : Inport  Port=4
  VTQD_CreepPrLoadEnable_flg : Inport  Port=5
  VTQD_CreepEnable_flg : Inport  Port=6
  VTQD_RrPreloadTq_Nm : Inport  Port=7
  VTQD_FrPreloadTq_Nm : Inport  Port=8
  VTQD_PreLoadHold_flg : Inport  Port=9
  VTQR_FrTqZeroTransLowBound_Nm : Inport  Port=10
  VTQR_RrTqZeroTransLowBound_Nm : Inport  Port=11
  AND10 : Logic  AllPortsSameDT=off  OutDataTypeStr=boolean
  AND15 : Logic  Inputs=3  AllPortsSameDT=off  OutDataTypeStr=boolean
  AND16 : Logic  Inputs=3  AllPortsSameDT=off  OutDataTypeStr=boolean
  AWD_Ratio : Subsystem  AncestorBlock=tqd/TQD/TorqueDemand/TorqueModule/TqDistribution/AWD_Ratio  TreatAsAtomicUnit=on
  Abs : Abs
  Abs1 : Abs
  Bus Selector : BusSelector  OutputSignals=task_time_s,VVMC_RearTqRatio_rat,VTQD_LimpHomeAct_flg,VINP_IVISnowModeCmd_flg,VVMC_ActLRSlideRate_pct,VVMC_ActRRSlideRate_pct,VTQD_ActAPSPosn_pct,VPMM_DrivetrainSelect_enum,VVMC_APSActive_flg,VINP_RrMotorAvailTq_Nm,VINP_RrRegenAvailTq_Nm,VINP_FrMotorAvailTq_Nm,VINP_FrRegenAvailTq_Nm
  Bus Selector1 : BusSelector  OutputSignals=VTQD_RrShaftSpd_rpm,VTQD_EVDriveMode_enum,VTQD_FrShaftSpd_rpm
  Bus Selector2 : BusSelector  OutputSignals=VTQD_EstVehWeightResult_kg,VTQD_FrontSlideRate_pct,VTQD_RearSlideRate_pct
  Bus Selector3 : BusSelector  OutputSignals=VTQD_DriverWhlTqDem_Nm,VTQD_CoordTqDem_Nm,VTQR_NoABSFEDUWhlTqReq_Nm,VTQR_NoABSREDUWhlTqReq_Nm
  Constant1 : Constant  Value=ENUM_DRIVETRAIN_RWD  VectorParams1D=off  SampleTime=-1
  Constant2 : Constant  Value=ENUM_DRIVETRAIN_AWD  VectorParams1D=off  SampleTime=-1
  Constant29 : Constant  Value=KTQD_AWDWhlTqRatioSW_flg
  Constant30 : Constant  Value=ENUM_DRIVEMODE_SPORT
  Constant31 : Constant  Value=ENUM_DRIVEMODE_NRM
  Constant32 : Constant  Value=ENUM_DRIVEMODE_ECO
  Constant33 : Constant  Value=ENUM_DRIVEMODE_SPORT
  Constant42 : Constant  Value=KTQD_NewWhlTqDistSW_flg  VectorParams1D=off  SampleTime=-1
  Constant43 : Constant  Value=KTQD_NewTotalCapTqSW_flg  VectorParams1D=off  SampleTime=-1
  Constant44 : Constant  Value=KTQD_NewPrelaodSW_flg  VectorParams1D=off  SampleTime=-1
  Constant45 : Constant  Value=KTQD_NewWhlTqDistSW_flg  VectorParams1D=off  SampleTime=-1
  Constant46 : Constant  Value=KTQD_NewTotalCapTqSW_flg  VectorParams1D=off  SampleTime=-1
  Constant47 : Constant  Value=KTQD_NewPrelaodSW_flg  VectorParams1D=off  SampleTime=-1
  Delay : Delay  DelayLength=1  InitialCondition=single(0)
      settings: AttributesFormatString=%<InitialCondition>
  Delay1 : Delay  DelayLength=1  InitialCondition=single(0)
      settings: AttributesFormatString=%<InitialCondition>
  Equal{1..2,14..17} (6 alike) : RelationalOperator  Operator===  OutDataTypeStr=boolean  RndMeth=Simplest
  FWD_Ratio : tqd/TQD/TorqueDemand/TorqueModule/TqDistribution/FWD_Ratio  SystemSampleTime=-1  VariantActivationTime=update diagram  Latency=0  AutoFrameSizeCalculation=off
  If : If  NumInputs=2  IfExpression=u1 ~= 0  ElseIfExpressions=u2 ~= 0
  LiuzgSwitch{1..3,13} (4 alike) : Switch  Criteria=u2 ~= 0
      settings: AttributesFormatString=<%<Criteria>>
  MTQD_AWDLoadTrqnsGain_Z_c : Lookup_n-D  BreakpointsForDimension1=ATQD_AWDLoadTrqnsGain_Y_pct  BreakpointsForDimension2=ATQD_AWDLoadTrqnsGain_X_kg  Table=MTQD_AWDLoadTrqnsGain_Z_c  ExtrapMethod=Clip  InternalRulePriority=Speed  RndMeth=Simplest  InputSameDT=on
      settings: InputPortMap=u0,u1
  MTQD_CreepRrTqSpRat_Z_rat : Lookup_n-D  BreakpointsForDimension1=ATQD_CreepRrTqSpRat_Y_Nm  BreakpointsForDimension2=ATQD_CreepRrTqSpRat_X_rpm  Table=MTQD_CreepRrTqSpRat_Z_rat  ExtrapMethod=Clip  InternalRulePriority=Speed  RndMeth=Simplest  InputSameDT=on
      settings: InputPortMap=u0,u1
  MTQD_ECORrEDUSpRat_Z_rat : Lookup_n-D  BreakpointsForDimension1=ATQD_NRMRrEDUSpRat_Y_Nm  BreakpointsForDimension2=ATQD_NRMRrEDUSpRat_X_rpm  Table=MTQD_ECORrEDUSpRat_Z_rat  ExtrapMethod=Clip  InternalRulePriority=Speed  RndMeth=Simplest  InputSameDT=on
      settings: InputPortMap=u0,u1
  "MTQD_NRMRrEDUSpRat_Z_rat  " : Lookup_n-D  BreakpointsForDimension1=ATQD_NRMRrEDUSpRat_Y_Nm  BreakpointsForDimension2=ATQD_NRMRrEDUSpRat_X_rpm  Table=MTQD_NRMRrEDUSpRat_Z_rat  ExtrapMethod=Clip  InternalRulePriority=Speed  RndMeth=Simplest  InputSameDT=on
      settings: InputPortMap=u0,u1
  MTQD_NRMRrEDUSpRat_Z_rat  1 : Lookup_n-D  BreakpointsForDimension1=ATQD_NRMRrEDUSpRat_Y_Nm  BreakpointsForDimension2=ATQD_NRMRrEDUSpRat_X_rpm  Table=MTQD_NRMRrEDUSpRat_Z_rat  ExtrapMethod=Clip  InternalRulePriority=Speed  RndMeth=Simplest  InputSameDT=on
      settings: InputPortMap=u0,u1
  MTQD_RockModePedTqFr_Z_Nm : Lookup_n-D  BreakpointsForDimension1=ATQD_RockModePedTqFr_Y_rpm  BreakpointsForDimension2=ATQD_RockModePedTqFr_X_pct  Table=MTQD_RockModePedTqFr_Z_Nm  InternalRulePriority=Speed  RndMeth=Simplest  InputSameDT=on
      settings: InputPortMap=u0,u1
  MTQD_RockModePedTqRr_Z_Nm : Lookup_n-D  BreakpointsForDimension1=ATQD_RockModePedTqFr_Y_rpm  BreakpointsForDimension2=ATQD_RockModePedTqFr_X_pct  Table=MTQD_RockModePedTqRr_Z_Nm  InternalRulePriority=Speed  RndMeth=Simplest  InputSameDT=on
      settings: InputPortMap=u0,u1
  MTQD_RrRatioWithFrSR_Z_rat : Lookup_n-D  BreakpointsForDimension1=ATQD_RrRatioWithFrSR_Y_rat  BreakpointsForDimension2=ATQD_RrRatioWithFrSR_X_pct  Table=MTQD_RrRatioWithFrSR_Z_rat  ExtrapMethod=Clip  UseLastTableValue=on  InternalRulePriority=Speed  RndMeth=Simplest  InputSameDT=on
      settings: InputPortMap=u0,u1
  MTQD_RrRatioWithRrSR_Z_rat : Lookup_n-D  BreakpointsForDimension1=ATQD_RrRatioWithFrSR_Y_rat  BreakpointsForDimension2=ATQD_RrRatioWithFrSR_X_pct  Table=MTQD_RrRatioWithRrSR_Z_rat  ExtrapMethod=Clip  UseLastTableValue=on  InternalRulePriority=Speed  RndMeth=Simplest  InputSameDT=on
      settings: InputPortMap=u0,u1
  MTQD_RrTqSRRateTs_Y_c : Lookup_n-D  NumberOfTableDimensions=1  BreakpointsForDimension1=ATQD_RrTqSRRateTs_X_pct  Table=MTQD_RrTqSRRateTs_Y_c  InternalRulePriority=Speed  RndMeth=Simplest  InputSameDT=on
  "MTQD_SPORTRrEDUSpRat_Z_rat " : Lookup_n-D  BreakpointsForDimension1=ATQD_NRMRrEDUSpRat_Y_Nm  BreakpointsForDimension2=ATQD_NRMRrEDUSpRat_X_rpm  Table=MTQD_SPORTRrEDUSpRat_Z_rat  ExtrapMethod=Clip  InternalRulePriority=Speed  RndMeth=Simplest  InputSameDT=on
      settings: InputPortMap=u0,u1
  MTQD_SnowMRrEDUSpRat_Z_rat : Lookup_n-D  BreakpointsForDimension1=ATQD_NRMRrEDUSpRat_Y_Nm  BreakpointsForDimension2=ATQD_NRMRrEDUSpRat_X_rpm  Table=MTQD_SnowMRrEDUSpRat_Z_rat  ExtrapMethod=Clip  InternalRulePriority=Speed  RndMeth=Simplest  InputSameDT=on
      settings: InputPortMap=u0,u1
  Max : MinMax  Function=max  Inputs=2
  Merge : Merge  Inputs=3
  Merge1 : Merge  Inputs=3
  New Torque Distribution : Subsystem  AncestorBlock=tqd/TQD/TorqueDemand/TorqueModule/TqDistribution/New Torque Distribution
  OR2 : Logic  Operator=OR  AllPortsSameDT=off  OutDataTypeStr=boolean
  Product : Product
  RWD_Ratio : tqd/TQD/TorqueDemand/TorqueModule/TqDistribution/RWD_Ratio  SystemSampleTime=-1  VariantActivationTime=update diagram  Latency=0  AutoFrameSizeCalculation=off
  Switch10 : Switch  Criteria=u2 > Threshold
  Switch15 : Switch  Criteria=u2 ~= 0
      settings: AttributesFormatString=%<Criteria>
  Switch16 : Switch  Criteria=u2 ~= 0
      settings: AttributesFormatString=%<Criteria>
  VTQD_FrEDUSpRat_rat : Outport
  VTQD_RrEDUSpRat_rat : Outport  Port=2
  VTQD_RockModePedTqFr_Nm : Outport  Port=3
  VTQD_RockModePedTqRr_Nm : Outport  Port=4
  VTQD_TMEnOutpTqSta_enum : Outport  Port=5
  VTQD_NewDistFrWhlTq_Nm : Outport  Port=6
  VTQD_NewDistRrWhlTq_Nm : Outport  Port=7
  wires:
  [task_time_s] -> AWD_Ratio/8(task_time_s)
  [VTQD_OrigRrDriverRatio_rat] -> AWD_Ratio/5(VTQD_OrigRrDriverRatio_rat)
  RWD_Ratio/1 -> [VTQD_FrRatio_RWD]  "VTQD_FrRatio_RWD"
  [VTQD_CreepRrTqSpRat_rat] -> AWD_Ratio/6(VTQD_CreepRrTqSpRat_rat)
  FWD_Ratio/2 -> [VTQD_RrRatio_FWD]  "VTQD_RrRatio_FWD"
  [VTQD_CreepEnable_flg] -> AWD_Ratio/4(VTQD_CreepEnable_flg)
  [VTQD_RrTqSRRateTs_c] -> AWD_Ratio/7(VTQD_RrTqSRRateTs_c)
  [VTQD_RrRatioWithRrSR_rat] -> AWD_Ratio/3(VTQD_RrRatioWithRrSR_rat)
  AWD_Ratio/2(VTQD_RrRatio_AWD) -> [VTQD_RrRatio_AWD]  "VTQD_RrRatio_AWD"
  If/1 -> RWD_Ratio/Action
  [VTQD_CreepPrLoadEnable_flg] -> AWD_Ratio/2(VTQD_CreepPrLoadEnable_flg)
  [VVMC_APSActive_flg] -> AWD_Ratio/1(VVMC_APSActive_flg)
  If/3 -> FWD_Ratio/Action
  FWD_Ratio/1 -> [VTQD_FrRatio_FWD]  "VTQD_FrRatio_FWD"
  Constant1/1 -> Equal1/2
  RWD_Ratio/2 -> [VTQD_RrRatio_RWD]  "VTQD_RrRatio_RWD"
  Constant2/1 -> Equal2/2
  [VPMM_DrivetrainSelect_enum] -> Equal2/1
  Equal2/1 -> If/2
  Equal1/1 -> If/1
  If/2 -> AWD_Ratio/Action
  [VPMM_DrivetrainSelect_enum] -> Equal1/1
  AWD_Ratio/1(VTQD_FrRatio_AWD) -> [VTQD_FrRatio_AWD]  "VTQD_FrRatio_AWD"
  Equal14/1 -> LiuzgSwitch1/2
  [VINP_IVISnowModeCmd_flg] -> LiuzgSwitch2/2
  [VVMC_ActLRSlideRate_pct] -> Abs/1
  [VTQD_RrShaftSpd_rpm] -> "MTQD_SPORTRrEDUSpRat_Z_rat "/2
  [VTQD_RrShaftSpd_rpm] -> MTQD_NRMRrEDUSpRat_Z_rat  1/2
  [VTQD_ActAPSPosn_pct] -> MTQD_RrTqSRRateTs_Y_c/1
  Equal17/1 -> OR2/2
  [VTQD_DriverWhlTqDem_Nm] -> MTQD_CreepRrTqSpRat_Z_rat/1
  [VTQD_RrShaftSpd_rpm] -> MTQD_CreepRrTqSpRat_Z_rat/2
  Equal16/1 -> OR2/1
  LiuzgSwitch1/1 -> LiuzgSwitch3/3
  [VTQD_AWDLoadTrqnsGain_c] -> Product/2
  [VTQD_EstVehWeightResult_kg] -> MTQD_AWDLoadTrqnsGain_Z_c/2
  Constant29/1 -> AND10/2
  [VTQD_EVDriveMode_enum] -> Equal15/1
  [VTQD_EVDriveMode_enum] -> Equal14/1
  [VTQD_RrShaftSpd_rpm] -> "MTQD_NRMRrEDUSpRat_Z_rat  "/2
  MTQD_ECORrEDUSpRat_Z_rat/1 -> LiuzgSwitch3/1
  MTQD_CreepRrTqSpRat_Z_rat/1 -> [VTQD_CreepRrTqSpRat_rat]  "VTQD_CreepRrTqSpRat_rat"
  LiuzgSwitch2/1 -> LiuzgSwitch13/3
  Constant32/1 -> Equal15/2
  MTQD_NRMRrEDUSpRat_Z_rat  1/1 -> LiuzgSwitch1/3
  [VTQD_DriverWhlTqDem_Nm] -> MTQD_NRMRrEDUSpRat_Z_rat  1/1
  [VTQD_RrShaftSpd_rpm] -> MTQD_ECORrEDUSpRat_Z_rat/2
  Constant31/1 -> Equal17/2
  "MTQD_SPORTRrEDUSpRat_Z_rat "/1 -> LiuzgSwitch1/1
  [VTQD_EVDriveMode_enum] -> Equal16/1
  OR2/1 -> AND10/1
  "MTQD_NRMRrEDUSpRat_Z_rat  "/1 -> LiuzgSwitch13/1
  [VTQD_DriverWhlTqDem_Nm] -> MTQD_ECORrEDUSpRat_Z_rat/1
  MTQD_RrTqSRRateTs_Y_c/1 -> [VTQD_RrTqSRRateTs_c]  "VTQD_RrTqSRRateTs_c"
  Equal15/1 -> LiuzgSwitch3/2
  Constant33/1 -> Equal14/2
  MTQD_AWDLoadTrqnsGain_Z_c/1 -> [VTQD_AWDLoadTrqnsGain_c]  "VTQD_AWDLoadTrqnsGain_c"
  LiuzgSwitch13/1 -> Product/1
  [VTQD_LimpHomeAct_flg] -> LiuzgSwitch13/2
  [VTQD_EVDriveMode_enum] -> Equal17/1
  [VVMC_RearTqRatio_rat] -> Switch10/1
  Max/1 -> MTQD_AWDLoadTrqnsGain_Z_c/1  "VTQD_AWDLoadTrqnsGain_pct"
  Constant30/1 -> Equal16/2
  [VTQD_SnowMRrEDUSpRat_rat] -> LiuzgSwitch2/1
  Product/1 -> Switch10/3
  LiuzgSwitch3/1 -> LiuzgSwitch2/3
  AND10/1 -> Switch10/2
  Abs/1 -> Max/1
  Abs1/1 -> Max/2
  Switch10/1 -> [VTQD_OrigRrDriverRatio_rat]  "VTQD_OrigRrDriverRatio_rat"
  [VTQD_DriverWhlTqDem_Nm] -> "MTQD_SPORTRrEDUSpRat_Z_rat "/1
  [VTQD_DriverWhlTqDem_Nm] -> "MTQD_NRMRrEDUSpRat_Z_rat  "/1
  [VVMC_ActRRSlideRate_pct] -> Abs1/1
  [VTQD_DriverWhlTqDem_Nm] -> MTQD_SnowMRrEDUSpRat_Z_rat/1
  MTQD_SnowMRrEDUSpRat_Z_rat/1 -> [VTQD_SnowMRrEDUSpRat_rat]  "VTQD_SnowMRrEDUSpRat_rat"
  [VTQD_RrShaftSpd_rpm] -> MTQD_SnowMRrEDUSpRat_Z_rat/2
  MTQD_RrRatioWithFrSR_Z_rat/1 -> [VTQD_RrRatioWithFrSR_rat]  "VTQD_RrRatioWithFrSR_rat"
  [VTQD_FrontSlideRate_pct] -> MTQD_RrRatioWithFrSR_Z_rat/2
  [VTQD_RearSlideRate_pct] -> MTQD_RrRatioWithRrSR_Z_rat/2
  MTQD_RockModePedTqRr_Z_Nm/1 -> [VTQD_RockModePedTqRr_Nm]  "VTQD_RockModePedTqRr_Nm"
  [VTQD_FrShaftSpd_rpm] -> MTQD_RockModePedTqFr_Z_Nm/1
  [VTQD_RrRatioWithFrSR_rat] -> MTQD_RrRatioWithRrSR_Z_rat/1
  [VTQD_ActAPSPosn_pct] -> MTQD_RockModePedTqFr_Z_Nm/2
  [VTQD_RrShaftSpd_rpm] -> MTQD_RockModePedTqRr_Z_Nm/1
  [VTQD_OrigRrDriverRatio_rat] -> MTQD_RrRatioWithFrSR_Z_rat/1
  [VTQD_ActAPSPosn_pct] -> MTQD_RockModePedTqRr_Z_Nm/2
  MTQD_RockModePedTqFr_Z_Nm/1 -> [VTQD_RockModePedTqFr_Nm]  "VTQD_RockModePedTqFr_Nm"
  MTQD_RrRatioWithRrSR_Z_rat/1 -> [VTQD_RrRatioWithRrSR_rat]  "VTQD_RrRatioWithRrSR_rat"
  BSCPIn_outputs/1 -> Bus Selector/1
  BSignalConvert_outputs/1 -> Bus Selector1/1
  BFunction_outputs/1 -> Bus Selector2/1
  BMain_outputs/1 -> Bus Selector3/1
  Bus Selector1/1 -> [VTQD_RrShaftSpd_rpm]  "<VTQD_RrShaftSpd_rpm>"
  Bus Selector/2 -> [VVMC_RearTqRatio_rat]  "<VVMC_RearTqRatio_rat>"
  Bus Selector1/2 -> [VTQD_EVDriveMode_enum]  "<VTQD_EVDriveMode_enum>"
  Bus Selector/3 -> [VTQD_LimpHomeAct_flg]  "<VTQD_LimpHomeAct_flg>"
  Bus Selector/4 -> [VINP_IVISnowModeCmd_flg]  "<VINP_IVISnowModeCmd_flg>"
  Bus Selector/5 -> [VVMC_ActLRSlideRate_pct]  "<VVMC_ActLRSlideRate_pct>"
  Bus Selector/6 -> [VVMC_ActRRSlideRate_pct]  "<VVMC_ActRRSlideRate_pct>"
  Bus Selector2/1 -> [VTQD_EstVehWeightResult_kg]  "<VTQD_EstVehWeightResult_kg>"
  Bus Selector/7 -> [VTQD_ActAPSPosn_pct]  "<VTQD_ActAPSPosn_pct>"
  Bus Selector2/2 -> [VTQD_FrontSlideRate_pct]  "<VTQD_FrontSlideRate_pct>"
  Bus Selector2/3 -> [VTQD_RearSlideRate_pct]  "<VTQD_RearSlideRate_pct>"
  Bus Selector1/3 -> [VTQD_FrShaftSpd_rpm]  "<VTQD_FrShaftSpd_rpm>"
  Bus Selector/8 -> [VPMM_DrivetrainSelect_enum]  "<VPMM_DrivetrainSelect_enum>"
  Bus Selector/9 -> [VVMC_APSActive_flg]  "<VVMC_APSActive_flg>"
  Bus Selector/1 -> [task_time_s]  "<task_time_s>"
  [VINP_FrRegenAvailTq_Nm] -> New Torque Distribution/10(VINP_FrRegenAvailTq_Nm)
  [VPMM_DrivetrainSelect_enum] -> New Torque Distribution/1(VPMM_DrivetrainSelect_enum)
  New Torque Distribution/4(VTQD_NewFrRatio_rat) -> [VTQD_NewFrRatio_rat]
  New Torque Distribution/2(VTQD_NewDistFrWhlTq_Nm) -> [VTQD_NewDistFrWhlTq_Nm]
  [VINP_RrMotorAvailTq_Nm] -> New Torque Distribution/7(VINP_RrMotorAvailTq_Nm)
  [VTQR_NoABSREDUWhlTqReq_Nm] -> Delay1/1
  [VTQR_RrTqZeroTransUpBound_Nm] -> New Torque Distribution/6(VTQR_RrTqZeroTransUpBound_Nm)
  [VTQD_PreLoadHold_flg] -> New Torque Distribution/13(VTQD_PreLoadHold_flg)
  [VTQD_FrPreloadTq_Nm] -> New Torque Distribution/12(VTQD_FrPreloadTq_Nm)
  [VTQR_NoABSFEDUWhlTqReq_Nm] -> Delay/1
  [VTQR_FrTqZeroTransLowBound_Nm] -> New Torque Distribution/4(VTQR_FrTqZeroTransLowBound_Nm)
  [VTQD_CoordTqDem_Nm] -> New Torque Distribution/2(VTQD_CoordTqDem_Nm)
  New Torque Distribution/5(VTQD_NewRrRatio_rat) -> [VTQD_NewRrRatio_rat]
  [VINP_FrMotorAvailTq_Nm] -> New Torque Distribution/9(VINP_FrMotorAvailTq_Nm)
  [VINP_RrRegenAvailTq_Nm] -> New Torque Distribution/8(VINP_RrRegenAvailTq_Nm)
  [VTQD_RrPreloadTq_Nm] -> New Torque Distribution/11(VTQD_RrPreloadTq_Nm)
  New Torque Distribution/3(VTQD_NewDistRrWhlTq_Nm) -> [VTQD_NewDistRrWhlTq_Nm]
  Bus Selector/10 -> [VINP_RrMotorAvailTq_Nm]  "<VINP_RrMotorAvailTq_Nm>"
  Bus Selector/11 -> [VINP_RrRegenAvailTq_Nm]  "<VINP_RrRegenAvailTq_Nm>"
  Bus Selector/12 -> [VINP_FrMotorAvailTq_Nm]  "<VINP_FrMotorAvailTq_Nm>"
  Bus Selector/13 -> [VINP_FrRegenAvailTq_Nm]  "<VINP_FrRegenAvailTq_Nm>"
  New Torque Distribution/1(VTQD_TMEnOutpTqSta_enum) -> [VTQD_TMEnOutpTqSta_enum]
  AND16/1 -> Switch16/2
  Constant47/1 -> AND16/1
  [VTQD_FrRatio_AWD] -> Merge/3
  [VTQD_NewRrRatio_rat] -> Switch16/1
  AND15/1 -> Switch15/2
  [VTQD_FrRatio_FWD] -> Merge/1
  Constant45/1 -> AND16/3
  Switch15/1 -> [VTQD_FrEDUSpRat_rat]  "VTQD_FrEDUSpRat_rat"
  Merge/1 -> Switch15/3
  [VTQD_RrRatio_RWD] -> Merge1/2
  Constant43/1 -> AND15/2
  Switch16/1 -> [VTQD_RrEDUSpRat_rat]  "VTQD_RrEDUSpRat_rat"
  [VTQD_FrRatio_RWD] -> Merge/2
  Constant42/1 -> AND15/3
  Constant44/1 -> AND15/1
  [VTQD_NewFrRatio_rat] -> Switch15/1
  [VTQD_RrRatio_AWD] -> Merge1/3
  [VTQD_RrRatio_FWD] -> Merge1/1
  Constant46/1 -> AND16/2
  Merge1/1 -> Switch16/3
  Bus Selector3/1 -> [VTQD_DriverWhlTqDem_Nm]  "<VTQD_DriverWhlTqDem_Nm>"
  Bus Selector3/2 -> [VTQD_CoordTqDem_Nm]  "<VTQD_CoordTqDem_Nm>"
  VTQD_CreepPrLoadEnable_flg/1 -> [VTQD_CreepPrLoadEnable_flg]
  VTQD_CreepEnable_flg/1 -> [VTQD_CreepEnable_flg]
  VTQD_RrPreloadTq_Nm/1 -> [VTQD_RrPreloadTq_Nm]
  VTQD_FrPreloadTq_Nm/1 -> [VTQD_FrPreloadTq_Nm]
  VTQD_PreLoadHold_flg/1 -> [VTQD_PreLoadHold_flg]
  [VTQD_FrEDUSpRat_rat] -> VTQD_FrEDUSpRat_rat/1
  [VTQD_RrEDUSpRat_rat] -> VTQD_RrEDUSpRat_rat/1
  [VTQD_RockModePedTqFr_Nm] -> VTQD_RockModePedTqFr_Nm/1
  [VTQD_RockModePedTqRr_Nm] -> VTQD_RockModePedTqRr_Nm/1
  [VTQD_TMEnOutpTqSta_enum] -> VTQD_TMEnOutpTqSta_enum/1
  [VTQD_NewDistFrWhlTq_Nm] -> VTQD_NewDistFrWhlTq_Nm/1
  [VTQD_NewDistRrWhlTq_Nm] -> VTQD_NewDistRrWhlTq_Nm/1
  VTQR_FrTqZeroTransLowBound_Nm/1 -> [VTQR_FrTqZeroTransLowBound_Nm]
  VTQR_RrTqZeroTransLowBound_Nm/1 -> [VTQR_RrTqZeroTransUpBound_Nm]
  Delay/1 -> New Torque Distribution/3(VTQR_NoABSFEDUWhlTqReq_Nm)
  Delay1/1 -> New Torque Distribution/5(VTQR_NoABSREDUWhlTqReq_Nm)
  Bus Selector3/3 -> [VTQR_NoABSFEDUWhlTqReq_Nm]  "<VTQR_NoABSFEDUWhlTqReq_Nm>"
  Bus Selector3/4 -> [VTQR_NoABSREDUWhlTqReq_Nm]  "<VTQR_NoABSREDUWhlTqReq_Nm>"
